simulink model "SRF_PLL"  (R2020a)
settings: Solver=FixedStepAuto  StartTime=0.0  StopTime=0.1  FixedStep=1e-6  RelTol=1e-3
libraries: eeTransforms x1, simulink x1, mcbcontrolslib x1, powerlib x1
settings Model: Creator=Administrator  LastModifiedBy=Administrator

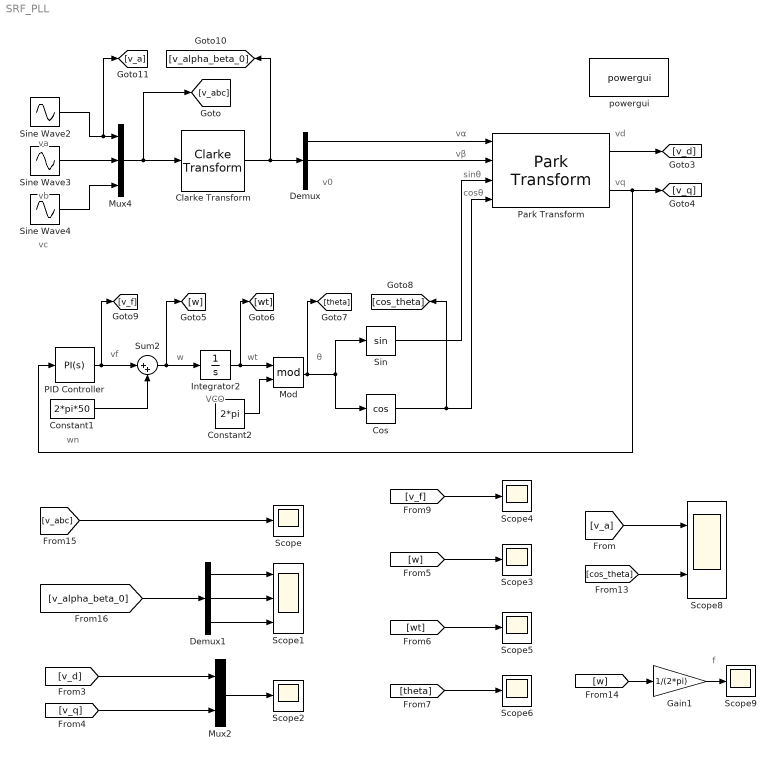
== system SRF_PLL ==
  note: v0
  note: VCO
  note: vq
  note: f
  note: wt
  note: w
  note: vd
  note: θ
  note: cosθ
  note: vα
  note: va
  note: wn
  note: vf
  note: sinθ
  note: vβ
  note: vb
  note: vc
  Clarke Transform : eeTransforms/Clarke Transform  PowerInvariant=off
      settings: SourceProductBaseCode=PS
  Constant1 : Constant  Value=2*pi*50
  Constant2 : Constant  Value=2*pi
  Cos : Trigonometry  Operator=cos
  Demux : Demux  Outputs=3
  Demux1 : Demux  Outputs=3
  Gain1 : Gain  Gain=1/(2*pi)
  Integrator2 : Integrator
  Mod : Math  Operator=mod  SaturateOnIntegerOverflow=on
  Mux2 : Mux  Inputs=2
  Mux4 : Mux  Inputs=3
  PID Controller : simulink/Continuous/PID Controller  Controller=PI  Form=Parallel  TimeDomain=Continuous-time  UseExternalTs=off  SampleTime=-1  IntegratorMethod=Forward Euler  FilterMethod=Forward Euler  ControllerParametersSource=internal  P=20  I=0.1  D=0  UseFilter=on  N=100  TunerSelectOption=Transfer Function Based (PID Tuner App)  InitialConditionSource=internal  InitialConditionForIntegrator=0  InitialConditionForFilter=0  DifferentiatorICPrevScaledInput=0  ExternalReset=none  TrackingMode=off  Kt=1  LimitOutput=off  UpperSaturationLimit=inf  LowerSaturationLimit=-inf  LinearizeAsGain=on  AntiWindupMode=none  Kb=1  POutMin=[]  POutMax=[]  IOutMin=[]  IOutMax=[]  DOutMin=[]  DOutMax=[]  NOutMin=[]  NOutMax=[]  SumOutMin=[]  SumOutMax=[]  SaturationOutMin=[]  SaturationOutMax=[]  PParamMin=[]  PParamMax=[]  IParamMin=[]  IParamMax=[]  DParamMin=[]  DParamMax=[]  NParamMin=[]  NParamMax=[]  KbParamMin=[]  KbParamMax=[]  KtParamMin=[]  KtParamMax=[]  KbOutMin=[]  KbOutMax=[]  KtOutMin=[]  KtOutMax=[]  IntegratorOutMin=[]  IntegratorOutMax=[]  FilterOutMin=[]  FilterOutMax=[]  SumI1OutMin=[]  SumI1OutMax=[]  SumI2OutMin=[]  SumI2OutMax=[]  SumI3OutMin=[]  SumI3OutMax=[]  SumI4OutMin=[]  SumI4OutMax=[]  SumDOutMin=[]  SumDOutMax=[]  DifferentiatorOutMin=[]  DifferentiatorOutMax=[]  FilterDiffOutCoefMin=[]  FilterDiffOutCoefMax=[]  ReciprocalOutMin=[]  ReciprocalOutMax=[]  SumDenOutMin=[]  SumDenOutMax=[]  SumNumOutMin=[]  SumNumOutMax=[]  DivideOutMin=[]  DivideOutMax=[]  UdiffTsProdOutMin=[]  UdiffTsProdOutMax=[]  NTsProdOutMin=[]  NTsProdOutMax=[]  UintegralTsProdOutMin=[]  UintegralTsProdOutMax=[]  UngainTsProdOutMin=[]  UngainTsProdOutMax=[]  IntegratorContinuousStateAttributes=''  IntegratorStateMustResolveToSignalObject=off  IntegratorRTWStateStorageClass=Auto  FilterContinuousStateAttributes=''  FilterStateMustResolveToSignalObject=off  FilterRTWStateStorageClass=Auto  ParallelPVariant=InternalParameters  IdealPVariant=Disabled  IVariant=InternalParameters  DVariant=Disabled  IntegratorVariant=Continuous  SatVariant=Disabled  AWVariant=Passthrough  PCopyVariant=Disabled  TRVariant=Disabled  FdbkBlocksVariant=Forward  IdealPFdbkVariant=Disabled  SatFdbkVariant=Disabled  DerivativeFilterVariant=Disabled  NVariant=Disabled  NCopyVariant=Disabled_SignalSpec  FilterICVariant=Disabled  IntegratorICVariant=InternalICs  ExternalResetVariant=Disabled  TRSumVariant=Passthrough  SumFdbkVariant=Disabled  SumVariant=Sum_PI  TsampFilterVariant=InternalTs  TsampNgainVariant=Passthrough  TsampIntegralVariant=Passthrough
  Park Transform : mcbcontrolslib/Park Transform  AxisAlignment=D-axis
      settings: SourceProductBaseCode=MT
  Scope{,2..6,9} (7 alike) : Scope
  Scope1 : Scope  NumInputPorts=3
  Scope8 : Scope  NumInputPorts=2
  Sin : Trigonometry
  Sine Wave2 : Sin  Amplitude=311  Frequency=2*3.1415926*50  Phase=3.1415926/2  SampleTime=0
  Sine Wave3 : Sin  Amplitude=311  Frequency=2*3.1415926*50  Phase=3.1415926/2-3.1415926*2/3  SampleTime=0
  Sine Wave4 : Sin  Amplitude=311  Frequency=2*3.1415926*50  Phase=3.1415926/2+3.1415926*2/3  SampleTime=0
  Sum2 : Sum  Inputs=|++
  powergui : powerlib/powergui  Priority=1  SimulationMode=Discrete  SampleTime=1e-6  frequency=60  Iterations=50  frequencyindice=60  Pbase=100e6  ErrMax=1e-4  UnitsV=kV  UnitsW=MW  buscounter=0  FunctionMessages=off  echomessages=off  EnableUseOfTLC=off  CurrentSourceSwitches=off  DisableSnubberDevices=off  DisableRonSwitches=off  DisableVfSwitches=off  DisplayEquations=off  AutomaticDiscreteSolvers=off  SolverType=Tustin/Backward Euler (TBE)  Interpol=off  ExternalGateDelay=off  methode=off  Ts=100  x0status=blocks  SPID=on  SwTol=0  HookPort=off  NonlinearTolerance=1e-4  nMaxIteration=100  ContinueOnMaxIteration=off  RestoreLinks=warning  ResistiveCurrentMeasurement=off  Frange=[0:2:500]  Ylog=off  Xlog=on  ShowGrid=off  save=off  variable=ZData  structure=0  ZoomFFT=off  StartTime=0.0  cycles=1  DisplayStyle=1  fundamental=60  FreqAxis=off  MaxFrequency=1000  frequencyindicesteady=1  RmsSteady=1  display=off
  wires:
  Constant2/1 -> Mod/2
  Constant1/1 -> Sum2/2
  [w] -> Gain1/1
  Gain1/1 -> Scope9/1
  [cos_theta] -> Scope8/2
  [v_d] -> Mux2/1
  [v_a] -> Scope8/1
  Mux2/1 -> Scope2/1
  Sum2/1 -> [w], Integrator2/1
  Park Transform/2 -> [v_q], PID Controller/1
  Cos/1 -> [cos_theta], Park Transform/4
  Integrator2/1 -> [wt], Mod/1
  Sin/1 -> Park Transform/3
  PID Controller/1 -> [v_f], Sum2/1
  [wt] -> Scope5/1
  [v_f] -> Scope4/1
  [v_q] -> Mux2/2
  [theta] -> Scope6/1
  [w] -> Scope3/1
  Mod/1 -> [theta], Cos/1, Sin/1
  Park Transform/1 -> [v_d]
  Sine Wave3/1 -> Mux4/2
  Sine Wave2/1 -> [v_a], Mux4/1
  Sine Wave4/1 -> Mux4/3
  Mux4/1 -> [v_abc], Clarke Transform/1
  Clarke Transform/1 -> [v_alpha_beta_0], Demux/1
  Demux/1 -> Park Transform/1
  Demux/2 -> Park Transform/2
  [v_abc] -> Scope/1
  [v_alpha_beta_0] -> Demux1/1
  Demux1/1 -> Scope1/1
  Demux1/2 -> Scope1/2
  Demux1/3 -> Scope1/3
